simulink model "TwoTanks"  (R2020a)
settings: Solver=VariableStepAuto  StartTime=0.0  StopTime=250  RelTol=1e-3
values from neighbouring files (symbols this model uses):
  D = 4    [load_data.m]
  Pump = 2    [load_data.m]
settings Model: Creator=lydialagorga  LastModifiedBy=lydialagorga

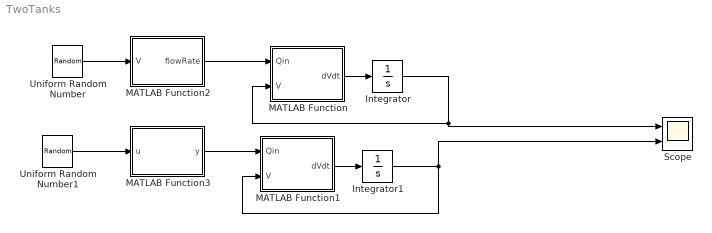
== system TwoTanks ==
  Integrator : Integrator  LimitOutput=on  UpperSaturationLimit=Inf  LowerSaturationLimit=0
  Integrator1 : Integrator  LimitOutput=on  UpperSaturationLimit=55  LowerSaturationLimit=0
  MATLAB Function : MATLAB Function  TreatAsAtomicUnit=on
  MATLAB Function1 : MATLAB Function  TreatAsAtomicUnit=on
  MATLAB Function2 : MATLAB Function  TreatAsAtomicUnit=on
  MATLAB Function3 : MATLAB Function  TreatAsAtomicUnit=on
  Scope : Scope  NumInputPorts=2
  Uniform Random Number : UniformRandomNumber  Minimum=2  Maximum=8  SampleTime=1
  Uniform Random Number1 : UniformRandomNumber  Minimum=2  Maximum=8  SampleTime=1
  wires:
  Integrator/1 -> MATLAB Function/2(V), Scope/1
  MATLAB Function/1(dVdt) -> Integrator/1
  Uniform Random Number/1 -> MATLAB Function2/1(V)
  Uniform Random Number1/1 -> MATLAB Function3/1(u)
  MATLAB Function1/1(dVdt) -> Integrator1/1
  Integrator1/1 -> Scope/2, MATLAB Function1/2(V)
  MATLAB Function3/1(y) -> MATLAB Function1/1(Qin)
  MATLAB Function2/1(flowRate) -> MATLAB Function/1(Qin)

== matlab function TwoTanks/MATLAB Function1 ==
  data: Qin input; dVdt output; V input; D parameter; Pump parameter
function dVdt = tank(Qin, V, D, Pump)
%Qout = Pump;
if V > 50.6
    Qout = Qin;
end
tankXA = pi*(4*D^2); %cross section area in m^2
height = V/tankXA; %height of fluid in tank m
Qout = sqrt(height);

dVdt = Qin - Qout; % rate of change of tank volume

== matlab function TwoTanks/MATLAB Function ==
  data: Qin input; dVdt output; V input; D parameter; Pump parameter
function dVdt = tank(Qin, V, D, Pump)
Qout = Pump;
if V > 220
    Qout = Qin;
end
%tankXA = pi*(4*D^2); %cross section area in m^2
%height = V/tankXA; %height of fluid in tank m

dVdt = Qin - Qout; % rate of change of tank volume

== matlab function TwoTanks/MATLAB Function2 ==
  data: V input; flowRate output
function flowRate = pipeFlow(V)
%things that determine pipe flow :) :P ;P  ;,,,)
flowRate = u;

== matlab function TwoTanks/MATLAB Function3 ==
  data: u input; y output
function y = fcn(u)

y = u;
